simulink model "MOT_CTRL_CTRL_FUN_003"  (R2025a)
settings: Solver=FixedStepAuto  StartTime=0.0  StopTime=10.0  FixedStep=1e-4  RelTol=1e-3
settings Model: DataDictionary=PIDControl.sldd  Creator=tecnicomcbti  LastModifiedBy=tecnicomcbti
settings SolverCC: ConcurrentTasks=on  AutoInsertRateTranBlk=on
settings DebuggingCC: UnderspecifiedInitializationDetection=Classic  MergeDetectMultiDrivingBlocksExec=none
settings ModelReferenceCC: PropagateSignalLabelsOutOfModel=off

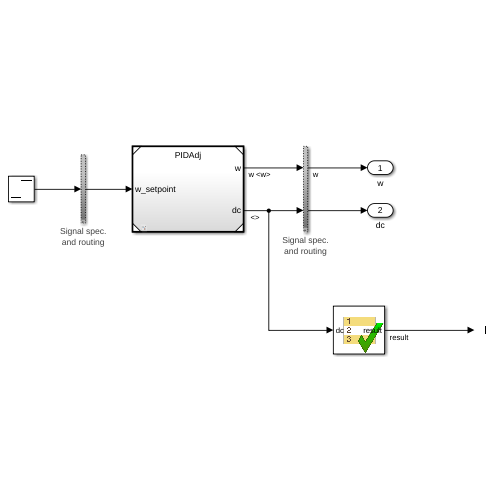
[thumbnail: Simulink's stored preview of the top-level diagram]
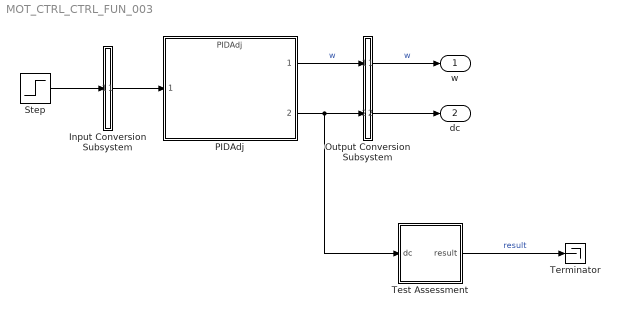
== system MOT_CTRL_CTRL_FUN_003 ==
  Input Conversion Subsystem : Subsystem  Tag=__SLT_ICS__  Description=|
      | Signal spec.
      | and routing
      settings: AttributesFormatString=%<Description>
  Output Conversion Subsystem : Subsystem  Tag=__SLT_OCS__  Description=|
      | Signal spec.
      | and routing
      settings: AttributesFormatString=%<Description>
  PIDAdj : ModelReference  ModelNameDialog=PIDAdj  SimulationMode=Normal  ModelReferenceVersion=1.17
  Step : Step  After=6000*pi/30  SampleTime=0
  Terminator : Terminator
  Test Assessment : Test Sequence  TreatAsAtomicUnit=on
  w : Outport
  dc : Outport  Port=2
  wires:
  Step/1 -> Input Conversion Subsystem/1(Inport_1)
  Output Conversion Subsystem/1(Outport_1) -> w/1  "w"
  Output Conversion Subsystem/2(Outport_2) -> dc/1
  Input Conversion Subsystem/1(Outport_1) -> PIDAdj/1
  PIDAdj/1 -> Output Conversion Subsystem/1(Inport_1)  "w"
  PIDAdj/2 -> Test Assessment/1(dc), Output Conversion Subsystem/2(Inport_2)
  Test Assessment/1(result) -> Terminator/1  "result"

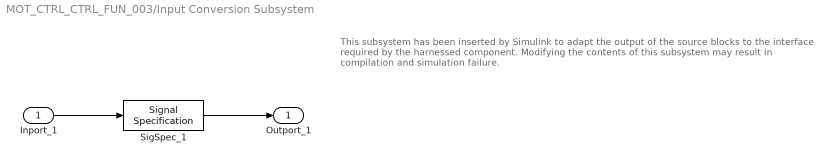
== system MOT_CTRL_CTRL_FUN_003/Input Conversion Subsystem ==
  note: This subsystem has been inserted by Simulink to adapt the output of the source blocks to the interface required by the harnessed component.
      |  Modifying the contents of this subsystem may result in compilation and simulation failure.
  Inport_1 : Inport
  SigSpec_1 : SignalSpecification  OutDataTypeStr=double  Dimensions=[1]  SampleTime=0.001
  Outport_1 : Outport
  wires:
  SigSpec_1/1 -> Outport_1/1
  Inport_1/1 -> SigSpec_1/1

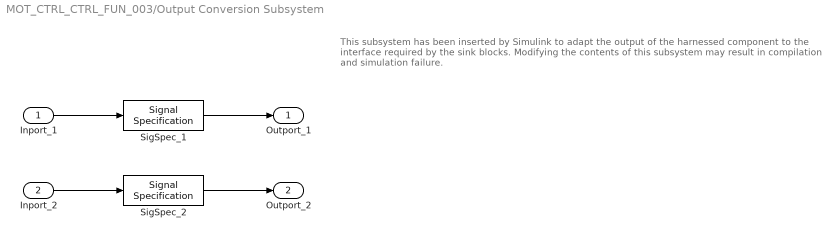
== system MOT_CTRL_CTRL_FUN_003/Output Conversion Subsystem ==
  note: This subsystem has been inserted by Simulink to adapt the output of the harnessed component to the interface required by the sink blocks.
      |  Modifying the contents of this subsystem may result in compilation and simulation failure.
  Inport_1 : Inport
  Inport_2 : Inport  Port=2
  SigSpec_1 : SignalSpecification  OutDataTypeStr=double  Dimensions=[1]
  SigSpec_2 : SignalSpecification  OutDataTypeStr=double  Dimensions=[1]  SampleTime=0.001
  Outport_1 : Outport
  Outport_2 : Outport  Port=2
  wires:
  Inport_1/1 -> SigSpec_1/1
  SigSpec_1/1 -> Outport_1/1
  Inport_2/1 -> SigSpec_2/1
  SigSpec_2/1 -> Outport_2/1

== stateflow chart MOT_CTRL_CTRL_FUN_003/Test Assessment ==
  state step_1
    if(dc>=0 && dc<=1)
    result=true;
    else
    result=false;
    end
  (default) -> step_1
  data: result output boolean; dc input
